simulink model "simpleLCMNode"  (Simulink 7.3)
settings: Solver=ode45  StartTime=0.0  StopTime=inf  FixedStep=.01  RelTol=1e-3
undefined symbols (not defined in the file or in its folder): getRobotName, simpleLCMNode_lcm_coder
libraries: robotlib x3
settings Model: Creator=russt  LastModifiedBy=russt
settings DebuggingCC: AlgebraicLoopMsg=none  SolverPrmCheckMsg=none  UnconnectedInputMsg=none  UnconnectedOutputMsg=none  UnconnectedLineMsg=none

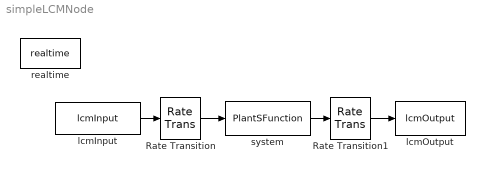
== system simpleLCMNode ==
  Rate Transition : RateTransition  OutPortSampleTimeOpt=Inherit
  Rate Transition1 : RateTransition  OutPortSampleTimeOpt=Inherit
  lcmInput : robotlib/lcmInput  channel=[lower(getRobotName(simpleLCMNode_lcm_coder)),'_u']  dim=1  decode_fcn=@(msg)decodeU(simpleLCMNode_lcm_coder,msg)  sample_time=0.01
  lcmOutput : robotlib/lcmOutput  channel=[lower(getRobotName(simpleLCMNode_lcm_coder)),'_xhat']  dim=2  encode_fcn=@(t,x)encodeX(simpleLCMNode_lcm_coder,t,x)  sample_time=0.01
  realtime : robotlib/realtime  sample_time=0.01
  system : M-S-Function  FunctionName=PlantSFunction  Parameters=simpleLCMNode_plantobj
  wires:
  lcmInput/1 -> Rate Transition/1
  system/1 -> Rate Transition1/1
  Rate Transition/1 -> system/1
  Rate Transition1/1 -> lcmOutput/1
